simulink library "HANcoder_STM32_Target2009b"  (R2023a)
settings: Solver=ode45  StartTime=0.0  StopTime=10.0  RelTol=1e-3  EnableMultiTasking=on
libraries: simulink x3
(part 5 of 7)

== system HANcoder_STM32_Target2009b/STM32-P405/Timer Inputs ==
  Quadrature Encoder Get : Subsystem  Tag=HANcoder_TARGET_STM32_P405  mask(Quadrature Encoder Inputs){moduleID=TIM3: PORTC PIN6 & PORTC PIN7 - 5V Tolerant, config=Floating, counterReset=off, tsamp=-1}
      mask prompts: moduleID "Quad encoder module"; config "Configuration"; counterReset "Show counter reset input"; tsamp "Sample time"
      mask help:
      | Function
      | ========
      | Reads the counter of the quadrature encoder module.
      |
      | Parameters
      | ==========
      | Quadrature encoder module:
      |   Selects the quadrature encoder module. The channel A and B signals of the
      |   encoder should be connected to the 2 input pins that belong to the module.
      |
      | Configuration:
      |   Determines if the input is floating or is connected to an internal
      |   pull-up or pull-down resistor.
      |
      | Show counter reset input:
      |   Configures if the input port for the counter reset should be shown.
      |
      |
      | Outport
      | ==========
      | 32-bit signed counter. The counter starts at zero and counts up or down
      | depending on the direction of the motor.
      mask init:
      | moduleIDInfoStr = sfcn_quad_encoder_get_mcb(3,moduleID, counterReset, config);
      settings: CopyFcn=sfcn_quad_encoder_get_chk();  MoveFcn=drawLogos
      mask Help: web('sfcn_quad_encoder_get.html');
      mask TypeOptions moduleID: TIM1: PORTA PIN8 & PORTA PIN9 - 5V Tolerant | TIM3: PORTC PIN6 & PORTC PIN7 - 5V Tolerant | TIM4: PORTB PIN6 & PORTB PIN7 - 5V Tolerant
      mask Callback moduleID: sfcn_quad_encoder_get_chk();
      mask TypeOptions config: Floating | Pullup | Pulldown
      mask Display: fprintf('Quad Encoder Get\n%s', moduleIDInfoStr);patch([135 141 141],[8 14 2],[1 0 0]);patch([143 143 149],[14 2 8],[0 0 0.35]);
  Timer Input Get : Subsystem  Tag=HANcoder_TARGET_STM32_P405  mask(Timer Input Get){pin=TIM1: Con. PA8 (PORTA PIN8) - 5V Tolerant, zeroHzTimeoutMs=2000, tsamp=-1}
      mask prompts: pin "Timer input pin"; zeroHzTimeoutMs "0 Hz detection time (ms)"; tsamp "Sample time"
      mask help:
      | Function
      | ========
      | Reads the information from a timer input pin.
      |
      | Parameters
      | ==========
      | Timer input pin:
      |   Selects the timer input pin.
      |
      | Zero Hz detection time:
      |   Determines after how many milliseconds since the last edge the 0 Hz
      |   detected output flag should go high.
      |
      | Outport
      | ==========
      | Frequency
      |   The last measured frequency on the pin in Hz.
      |
      | Duty cycle
      |   The last measured duty cycle on the pin as a % with a scaling factor of 100 for
      |   improved resolution. So 5000 = 50% for example.
      |
      | Edge count
      |   The number of edges that were detected on the input pin since startup.
      |
      | Edge timestamp
      |   A 32-bit timestamp value of the last edge. The timestamp is derived from an
      |   internal 32-bit free running counter that runs at 21 Mhz.
      |
      | 0 Hz detected
      |   A boolean flag that will go high if no edges were detected for the time specified
      |   as the zero Hz detection time. Upon the next edge the flag will go low again.
      mask init:
      | timeinPinIdInfoStr = sfcn_timein_get_mcb(3, pin, zeroHzTimeoutMs);
      settings: CopyFcn=sfcn_timein_get_chk();  MoveFcn=drawLogos
      mask Help: web('sfcn_timein_get.html');
      mask TypeOptions pin: TIM1: Con. PA8 (PORTA PIN8) - 5V Tolerant | TIM1: Con. UEXT-3 (PORTA PIN9) - 5V Tolerant | TIM1: Con. UEXT-4 (PORTA PIN10) - 5V Tolerant | TIM2: Con. PA1 (PORTA PIN1) - 5V Tolerant | TIM3: Con. PC6 (PORTC PIN6) - 5V Tolerant | TIM3: Con. PC7 (PORTC PIN7) - 5V Tolerant | TIM3: Con. PC8 (PORTC PIN8) - 5V Tolerant | TIM3: Con. PC9 (PORTC PIN9) - 5V Tolerant | TIM4: Con. UEXT-5 (PORTB PIN6) - 5V Tolerant | TIM4: Con. UEXT-6 (PORTB PIN7) - 5V Tolerant | TIM4: Con. PB8 (PORTB PIN8) - 5V Tolerant | TIM4: Con. PB9 (PORTB PIN9) - 5V Tolerant
      mask Callback pin: sfcn_timein_get_chk();
      mask Display:
      | fprintf('Timer Input Get\n%s', timeinPinIdInfoStr);
      | port_label('output', 1, 'Frequency');
      | port_label('output', 2, 'Duty cycle');
      | port_label('output', 3, 'Edge count');
      | port_label('output', 4, 'Edge state');
      | port_label('output', 5, 'Edge timestamp');
      | port_label('output', 6, 'Counter timestamp');
      | port_label('output', 7, '0 Hz detected');patch([250 256 256],[8 14 2],[1 0 0]);patch([258 258 264],[14 2 8],[0 0 0.35]);
  Timer Input IRQ : Subsystem  Tag=HANcoder_TARGET_STM32_P405  mask(Timer Input IRQ){pin=TIM1: Con. PA8 (PORTA PIN8) - 5V Tolerant}
      mask prompts: pin "Timer input pin"
      mask help:
      | Function
      | ========
      | Enables a function call subsystem to be connected that is executed on interrupt level
      | each time an edge change on the input pin was detected.
      |
      | Parameters
      | ==========
      | Timer input pin:
      |   Selects the timer input pin.
      |
      | Outport
      | =======
      | IRQ
      |   Allows connection of a function call subsystem.
      mask init:
      | timeinPinIdInfoStr = sfcn_timein_irq_mcb(3, pin);
      settings: CopyFcn=sfcn_timein_irq_chk();  MoveFcn=drawLogos
      mask Help: web('sfcn_timein_irq.html');
      mask TypeOptions pin: TIM1: Con. PA8 (PORTA PIN8) - 5V Tolerant | TIM1: Con. UEXT-3 (PORTA PIN9) - 5V Tolerant | TIM1: Con. UEXT-4 (PORTA PIN10) - 5V Tolerant | TIM2: Con. PA1 (PORTA PIN1) - 5V Tolerant | TIM3: Con. PC6 (PORTC PIN6) - 5V Tolerant | TIM3: Con. PC7 (PORTC PIN7) - 5V Tolerant | TIM3: Con. PC8 (PORTC PIN8) - 5V Tolerant | TIM3: Con. PC9 (PORTC PIN9) - 5V Tolerant | TIM4: Con. UEXT-5 (PORTB PIN6) - 5V Tolerant | TIM4: Con. UEXT-6 (PORTB PIN7) - 5V Tolerant | TIM4: Con. PB8 (PORTB PIN8) - 5V Tolerant | TIM4: Con. PB9 (PORTB PIN9) - 5V Tolerant
      mask Callback pin: sfcn_timein_irq_chk();
      mask Display: fprintf('Timer Input IRQ\n%s', timeinPinIdInfoStr);patch([250 256 256],[8 14 2],[1 0 0]);patch([258 258 264],[14 2 8],[0 0 0.35]);

== system HANcoder_STM32_Target2009b/STM32-P405/Timer Outputs ==
  Compare Event IRQ : Subsystem  Tag=HANcoder_TARGET_STM32_P405  mask(Compare Event IRQ){pin=TIM1: Con. PA8 (PORTA PIN8) - 5V Tolerant}
      mask prompts: pin "Timer output pin"
      mask help:
      | Function
      | ========
      | Enables a function call subsystem to be connected that is executed on interrupt
      | level each time an output compare event was triggered.
      |
      | Parameters
      | ==========
      | Timer Output Pin:
      |   Selects the timer channel.
      |
      | Outport
      | =======
      | IRQ
      |   Allows connection of a function call subsystem.
      mask init:
      | timeoutPinIdInfoStr = sfcn_timeout_event_irq_mcb(3, pin);
      settings: CopyFcn=sfcn_timeout_event_irq_chk();  MoveFcn=drawLogos
      mask Help: web('sfcn_timeout_event_irq.html');
      mask TypeOptions pin: TIM1: Con. PA8 (PORTA PIN8) - 5V Tolerant | TIM1: Con. UEXT-3 (PORTA PIN9) - 5V Tolerant | TIM1: Con. UEXT-4 (PORTA PIN10) - 5V Tolerant | TIM2: Con. PA1 (PORTA PIN1) - 5V Tolerant | TIM3: Con. PC6 (PORTC PIN6) - 5V Tolerant | TIM3: Con. PC7 (PORTC PIN7) - 5V Tolerant | TIM3: Con. PC8 (PORTC PIN8) - 5V Tolerant | TIM3: Con. PC9 (PORTC PIN9) - 5V Tolerant | TIM4: Con. UEXT-5 (PORTB PIN6) - 5V Tolerant | TIM4: Con. UEXT-6 (PORTB PIN7) - 5V Tolerant | TIM4: Con. PB8 (PORTB PIN8) - 5V Tolerant | TIM4: Con. PB9 (PORTB PIN9) - 5V Tolerant
      mask Callback pin: sfcn_timeout_event_irq_chk();
      mask Display: fprintf('Compare Event IRQ\n%s', timeoutPinIdInfoStr);patch([135 141 141],[8 14 2],[1 0 0]);patch([143 143 149],[14 2 8],[0 0 0.35]);
  Get Free Running Counter : Subsystem  Tag=HANcoder_TARGET_STM32_P405  mask(Get Free Running Counter){moduleID=TIM1, tsamp=-1}
      mask prompts: moduleID "Timer module"; tsamp "Sample time"
      mask help:
      | Function
      | ========
      | Reads the timer module's internal 16-bit free running counter value.
      |
      | Parameters
      | ==========
      | Timer Module:
      |   Selects the timer module.
      |
      | Outport
      | =======
      | 16-bit free running counter value.
      mask init:
      | moduleIDInfoStr = sfcn_timeout_getrunningcounter_mcb(3, moduleID);
      settings: MoveFcn=drawLogos
      mask Help: web('sfcn_timeout_getrunningcounter.html');
      mask TypeOptions moduleID: TIM1 | TIM2 | TIM3 | TIM4
      mask Display: fprintf('Get Free Running Counter\n%s', moduleIDInfoStr);patch([135 141 141],[8 14 2],[1 0 0]);patch([143 143 149],[14 2 8],[0 0 0.35]);
  Get Last Event Counter : Subsystem  Tag=HANcoder_TARGET_STM32_P405  mask(Get Last Event Counter){pin=TIM1: Con. PA8 (PORTA PIN8) - 5V Tolerant, tsamp=-1}
      mask prompts: pin "Timer output pin"; tsamp "Sample time"
      mask help:
      | Function
      | ========
      | Reads the timer channel's timestamp of the 16-bit free running counter
      | value at which the last output compare event occurred.
      |
      | Parameters
      | ==========
      | Timer Output Pin:
      |   Selects the timer channel.
      |
      | Outport
      | =======
      | 16-bit free running counter timestamp of the last output compare event.
      mask init:
      | timeoutPinIdInfoStr = sfcn_timeout_getlasteventcounter_mcb(3, pin);
      settings: MoveFcn=drawLogos
      mask Help: web('sfcn_timeout_getlasteventcounter.html');
      mask TypeOptions pin: TIM1: Con. PA8 (PORTA PIN8) - 5V Tolerant | TIM1: Con. UEXT-3 (PORTA PIN9) - 5V Tolerant | TIM1: Con. UEXT-4 (PORTA PIN10) - 5V Tolerant | TIM2: Con. PA1 (PORTA PIN1) - 5V Tolerant | TIM3: Con. PC6 (PORTC PIN6) - 5V Tolerant | TIM3: Con. PC7 (PORTC PIN7) - 5V Tolerant | TIM3: Con. PC8 (PORTC PIN8) - 5V Tolerant | TIM3: Con. PC9 (PORTC PIN9) - 5V Tolerant | TIM4: Con. UEXT-5 (PORTB PIN6) - 5V Tolerant | TIM4: Con. UEXT-6 (PORTB PIN7) - 5V Tolerant | TIM4: Con. PB8 (PORTB PIN8) - 5V Tolerant | TIM4: Con. PB9 (PORTB PIN9) - 5V Tolerant
      mask Display: fprintf('Get Last Event Counter\n%s', timeoutPinIdInfoStr);patch([135 141 141],[8 14 2],[1 0 0]);patch([143 143 149],[14 2 8],[0 0 0.35]);
  Output Compare Init : Subsystem  Tag=HANcoder_TARGET_STM32_P405  mask(Output Compare Init){moduleID=TIM1: PA8 & PA9 & PA10 & n/a, frequency=2000000, enableIRQoutput=off}
      mask prompts: moduleID "Timer module"; frequency "Frequency (free running counter) [Hz]"; enableIRQoutput "Enable IRQ output"
      mask help:
      | Function
      | ========
      | Initializes the timer module to allow output compare functionality on the
      | module's channels.
      |
      | Parameters
      | ==========
      | Timer Module:
      |   Selects the timer module.
      |
      | Frequency:
      |   Frequency at which the 16-bit free running counter counts.
      |
      | Enable IRQ output
      |   Controls whether or not the IRQ output is available.
      |
      | Outport
      | =======
      | IRQ
      |   Allows connection of a function call subsystem for the free running
      |   counter overflow event.
      mask init:
      | moduleIDInfoStr = sfcn_timeout_init_mcb(3, moduleID, frequency, enableIRQoutput);
      settings: CopyFcn=sfcn_timeout_init_chk();  MoveFcn=drawLogos
      mask Help: web('sfcn_timeout_init.html');
      mask TypeOptions moduleID: TIM1: PA8 & PA9 & PA10 & n/a | TIM2: n/a & PA1 & n/a & n/a | TIM3: PC6 & PC7 & PC8 & PC9 | TIM4: PB6 & PB7 & PC8 & PB9
      mask Callback moduleID: sfcn_timeout_init_chk();
      mask Display: fprintf('Output Compare Init\n%s', moduleIDInfoStr);patch([135 141 141],[8 14 2],[1 0 0]);patch([143 143 149],[14 2 8],[0 0 0.35]);
  Reset Free Running Counter : Subsystem  Tag=HANcoder_TARGET_STM32_P405  mask(Reset Free Running Counter){moduleID=TIM1}
      mask prompts: moduleID "Timer module"
      mask help:
      | Function
      | ========
      | Resets the value of the timer module's 16-bit free running counter back to
      | 0.
      |
      | Triggerport
      | ===========
      | Connect the port to a trigger source to execute the block only when necessary.
      mask init:
      | moduleIDInfoStr = sfcn_timeout_resetcounter_mcb(3, moduleID);
      settings: MoveFcn=drawLogos
      mask Help: web('sfcn_timeout_resetcounter.html');
      mask TypeOptions moduleID: TIM1 | TIM2 | TIM3 | TIM4
      mask Display: fprintf('Reset Free Running Counter\n%s', moduleIDInfoStr);patch([132 138 138],[8 14 2],[1 0 0]);patch([140 140 146],[14 2 8],[0 0 0.35]);
  Schedule Compare Event : Subsystem  Tag=HANcoder_TARGET_STM32_P405  mask(Schedule Compare Event){pin=TIM1: Con. PA8 (PORTA PIN8) - 5V Tolerant, tsamp=-1}
      mask prompts: pin "Timer output pin"; tsamp "Sample time"
      mask help:
      | Function
      | ========
      | Schedules the next output compare event. The first input determines the
      | value of the timer module's 16-bit free running counter when the event
      | should trigger. The second input determines the action that should
      | be taken on the timer channel's pin.
      |
      | Parameters
      | ==========
      | Timer output pin:
      |   Selects the timer channel's pin.
      |
      | Inport
      | ======
      | Counter
      |   Value of the timer module's 16-bit free running counter at which the
      |   event should trigger.
      |
      | Action
      |   Action to take on the channel's pin when the event triggers:
      |   0: set output pin to logic low.
      |   1: set output pin to logic high.
      |   2: invert logic state of the outpin pin.
      |   3: do nothing to the output pin.
      mask init:
      | timeoutPinIdInfoStr = sfcn_timeout_scheduleevent_mcb(3, pin);
      settings: MoveFcn=drawLogos
      mask Help: web('sfcn_timeout_scheduleevent.html');
      mask TypeOptions pin: TIM1: Con. PA8 (PORTA PIN8) - 5V Tolerant | TIM1: Con. UEXT-3 (PORTA PIN9) - 5V Tolerant | TIM1: Con. UEXT-4 (PORTA PIN10) - 5V Tolerant | TIM2: Con. PA1 (PORTA PIN1) - 5V Tolerant | TIM3: Con. PC6 (PORTC PIN6) - 5V Tolerant | TIM3: Con. PC7 (PORTC PIN7) - 5V Tolerant | TIM3: Con. PC8 (PORTC PIN8) - 5V Tolerant | TIM3: Con. PC9 (PORTC PIN9) - 5V Tolerant | TIM4: Con. UEXT-5 (PORTB PIN6) - 5V Tolerant | TIM4: Con. UEXT-6 (PORTB PIN7) - 5V Tolerant | TIM4: Con. PB8 (PORTB PIN8) - 5V Tolerant | TIM4: Con. PB9 (PORTB PIN9) - 5V Tolerant
      mask Display: fprintf('Schedule Compare Event\n%s', timeoutPinIdInfoStr);patch([135 141 141],[8 14 2],[1 0 0]);patch([143 143 149],[14 2 8],[0 0 0.35]);

== system HANcoder_STM32_Target2009b/STM32-P405/UART ==
  UART init : Subsystem  Tag=HANcoder_TARGET_STM32_P405  mask(UART init){channel=UART1: Con. UEXT-3 & Con. UEXT-4 (PA9 & PA10), baudrate=19200, databits=8, parity=none, stopbits=1, txbufsize=32, rxbufsize=32, useStatusOut=off}
      mask prompts: baudrate "Baudrate (bit/s)"; txbufsize "Transmit buffer size"; rxbufsize "Receive buffer size"; useStatusOut "Use status output"
      mask help:
      | Function
      | ==========
      | Initialized a UART channel.
      |
      | Parameters per channel
      | ======================
      | - Select channel
      | - Select baudrate
      | - Select number of databits
      | - Select parity
      | - Select number of stopbits
      | - Configure the size of the transmit buffer
      | - Configure the size of the reception buffer
      | - Enable/disable the status output port
      mask init:
      | uartChannelInfoStr = sfcn_uart_init_mcb(3, channel, baudrate, databits, parity, stopbits, txbufsize, rxbufsize, useStatusOut);
      settings: CopyFcn=sfcn_uart_init_chk();  MoveFcn=drawLogos
      mask Help: web('sfcn_uart_init.html')
      mask TypeOptions channel: UART1: Con. UEXT-3 & Con. UEXT-4 (PA9 & PA10) | UART2: SUB D9 (PA2 & PA3)
      mask Callback channel: sfcn_uart_init_chk();
      mask TypeOptions baudrate: 300 | 600 | 1200 | 2400 | 4800 | 9600 | 19200 | 38400 | 57600 | 115200
      mask TypeOptions databits: 8 | 9
      mask TypeOptions parity: none | even | odd
      mask TypeOptions stopbits: 1 | 2
      mask Display: fprintf('UART init\n%s', uartChannelInfoStr);patch([236 242 242],[8 14 2],[1 0 0]);patch([244 244 250],[14 2 8],[0 0 0.35]);
  UART receive : Subsystem  Tag=HANcoder_TARGET_STM32_P405  mask(UART receive){channel=UART1: Con. UEXT-3 & Con. UEXT-4 (PA9 & PA10), useStatusOut=off, tsamp=-1}
      mask prompts: useStatusOut "Use status outport"; tsamp "Sample time"
      mask help:
      | Function
      | ==========
      | Reads a byte from the UART reception buffer.
      |
      | Parameters per channel
      | ======================
      | - Select channel
      | - Select if the status output should be enabled.
      |
      | Outputs
      | =======
      | - The value of the receive byte.
      | - When the status output is 0, the reception buffer was empty.
      mask init:
      | uartChannelInfoStr = sfcn_uart_receive_mcb(3, channel, useStatusOut);
      settings: MoveFcn=drawLogos
      mask Help: web('sfcn_uart_receive.html')
      mask TypeOptions channel: UART1: Con. UEXT-3 & Con. UEXT-4 (PA9 & PA10) | UART2: SUB D9 (PA2 & PA3)
      mask Display: fprintf('UART receive\n%s', uartChannelInfoStr);patch([240 246 246],[8 14 2],[1 0 0]);patch([248 248 254],[14 2 8],[0 0 0.35]);
  UART receive buffer status : Subsystem  Tag=HANcoder_TARGET_STM32_P405  mask(UART receive buffer status){channel=UART1: Con. UEXT-3 & Con. UEXT-4 (PA9 & PA10), tsamp=-1}
      mask prompts: tsamp "Sample time"
      mask help:
      | Function
      | ==========
      | Obtains the number of received bytes that are currently stored in the
      | reception buffer.
      |
      | Parameters per channel
      | ======================
      | - Select channel
      |
      | Outputs
      | ======
      | - The number of bytes currently stored in the reception buffer.
      mask init:
      | uartChannelInfoStr = sfcn_uart_receive_size_mcb(3, channel);
      settings: MoveFcn=drawLogos
      mask Help: web('sfcn_uart_receive_size.html')
      mask TypeOptions channel: UART1: Con. UEXT-3 & Con. UEXT-4 (PA9 & PA10) | UART2: SUB D9 (PA2 & PA3)
      mask Display: fprintf('UART receive buffer status\n%s', uartChannelInfoStr);patch([245 251 251],[8 14 2],[1 0 0]);patch([253 253 259],[14 2 8],[0 0 0.35]);
  UART send : Subsystem  Tag=HANcoder_TARGET_STM32_P405  mask(UART send){channel=UART1: Con. UEXT-3 & Con. UEXT-4 (PA9 & PA10), useStatusOut=off, tsamp=-1}
      mask prompts: useStatusOut "Use status outport"; tsamp "Sample time"
      mask help:
      | Function
      | ==========
      | Transmits a byte on the UART communication interface.
      |
      | Parameters per channel
      | ======================
      | - Select channel
      | - Select if the status output should be enabled.
      |
      | Inputs
      | ======
      | - The byte to send
      |
      | Outputs
      | =======
      | - When the status output is 0, the byte could not be transmitted. Probably
      |   because the transmit buffer was configured too small.
      mask init:
      | uartChannelInfoStr = sfcn_uart_send_mcb(3, channel, useStatusOut);
      settings: MoveFcn=drawLogos
      mask Help: web('sfcn_uart_send.html')
      mask TypeOptions channel: UART1: Con. UEXT-3 & Con. UEXT-4 (PA9 & PA10) | UART2: SUB D9 (PA2 & PA3)
      mask Display: fprintf('UART send\n%s', uartChannelInfoStr);patch([245 251 251],[8 14 2],[1 0 0]);patch([253 253 259],[14 2 8],[0 0 0.35]);

== system HANcoder_STM32_Target2009b/STM32-P405/UDS ==
  UDS Get Key : Subsystem  Tag=HANcoder_TARGET_STM32_P405  mask(UDS Get Key){tsamp=-1}
      mask prompts: tsamp "Sample time"
      mask help:
      | Function
      | ==========
      | Reads the 32-bit key value that was received from the UDS tester.
      |
      | Outport
      | =======
      |  - Key value that was received from the UDS tester.
      mask init:
      | sfcn_uds_get_key_mcb();
      settings: MoveFcn=drawLogos
      mask Help: web('sfcn_uds_get_key.html');
      mask Display: fprintf('UDS Get Key');patch([65 71 71],[8 14 2],[1 0 0]);patch([73 73 79],[14 2 8],[0 0 0.35]);
  UDS Get Seed : Subsystem  Tag=HANcoder_TARGET_STM32_P405  mask(UDS Get Seed){tsamp=-1}
      mask prompts: tsamp "Sample time"
      mask help:
      | Function
      | ==========
      | Reads the 32-bit seed value to be used in the seed/key unlock sequence.
      |
      | Outport
      | =======
      |  - Seed value to be used in the seed/key unlock sequence.
      mask init:
      | sfcn_uds_get_seed_mcb();
      settings: MoveFcn=drawLogos
      mask Help: web('sfcn_uds_get_seed.html');
      mask Display: fprintf('UDS Get Seed');patch([65 71 71],[8 14 2],[1 0 0]);patch([73 73 79],[14 2 8],[0 0 0.35]);
  UDS Get Seed Event : Subsystem  Tag=HANcoder_TARGET_STM32_P405  mask(UDS Get Seed Event){}
      mask help:
      | Function
      | ========
      | A 'UDS Get Seed Event' block is needed when the parameter 'UDS seed/key
      | required' is set to TRUE (checked) in the 'UDS Init' block.
      |
      | This block has a function call output that gets triggered during a seed/key
      | sequence, when the UDS module needs a seed. The connected subsystem should
      | contain a 'UDS Set Seed' block to give the seed back to the UDS module.
      |
      | Outport
      | =======
      | Event
      |   Allows connection of a function call subsystem.
      mask init:
      | sfcn_uds_get_seed_event_mcb();
      settings: MoveFcn=drawLogos
      mask Help: web('sfcn_uds_get_seed_event.html');
      mask Display: fprintf('UDS Get Seed Event');patch([95 101 101],[8 14 2],[1 0 0]);patch([103 103 109],[14 2 8],[0 0 0.35]);
  UDS Init : Subsystem  Tag=HANcoder_TARGET_STM32_P405  mask(UDS Init){canChannel=CAN 1, canTxId=hex2dec('7E8'), canRxId=hex2dec('7E0'), tpBlockSize=4, tpSTmin=40, tpRxBuffSize=64, udsTxBuffSize=64, udsUseSeedKey=off}
      mask prompts: canChannel "CAN channel"; canTxId "CAN transmit ID"; canRxId "CAN receive ID"; tpBlockSize "TP blocksize"; tpSTmin "TP STmin"; tpRxBuffSize "TP reception buffer size"; udsTxBuffSize "UDS transmit buffer size"; udsUseSeedKey "UDS seed/key required"
      mask help:
      | Function
      | ==========
      | Initializes the Unified Diagnostic Services (UDS) communication module.
      |
      | Parameters
      | ==========
      | CAN channel: The CAN channel to communicate on
      | CAN transmit ID: CAN identifier for ECU to Tester
      | CAN receive ID: CAN identifier for Tester to ECU
      | TP blocksize: Number of CF's to receive before sending a FC
      | TP STmin: Min separation time (ms) expected between CF's
      | TP reception buffer size: Size of the buffer for TP receptions
      | UDS transmit buffer size: Size of the buffer for UDS/TP transmissions
      | UDS seed/key required: Requires a seed/key unlock sequence
      mask init:
      | sfcn_uds_init_mcb(canChannel, canTxId, canRxId, tpBlockSize, tpSTmin, tpRxBuffSize, udsTxBuffSize, udsUseSeedKey);
      settings: MoveFcn=drawLogos
      mask Help: web('sfcn_uds_init.html');
      mask TypeOptions canChannel: CAN 1 | CAN 2
      mask TypeOptions tpBlockSize: 1 | 2 | 3 | 4 | 5 | 6 | 7 | 8 | 9 | 10 | 11 | 12 | 13 | 14 | 15 | 16 | 17 | 18 | 19 | 20 | 21 | 22 | 23 | 24 | 25 | 26 | 27 | 28 | 29 | 30 | 31 | 32 | 33 | 34 | 35 | 36 | 37 | 38 | 39 | 40 | 41 | 42 | 43 | 44 | 45 | 46 | 47 | 48 | 49 | 50 | 51 | 52 | 53 | 54 | 55 | 56 | 57 | 58 | 59 | 60 | 61 | 62 | 63 | 64 | 65 | 66 | 67 | 68 | 69 | 70 | 71 | 72 | 73 | 74 | 75 | 76 | 77 | 78 | 79 | 80 | 81 | 82 | 83 | 84 | 85 | 86 | 87 | 88 | 89 | 90 | 91 | 92 | 93 | 94 | 95 | 96 | 97 | 98 | 99 | 100 | 101 | 102 | 103 | 104 | 105 | 106 | 107 | 108 | 109 | 110 | 111 | 112 | 113 | 114 | 115 | 116 | 117 | 118 | 119 | 120 | 121 | 122 | 123 | 124 | 125 | 126 | 127 | 128 | 129 | 130 | 131 | 132 | 133 | 134 | 135 | 136 | 137 | 138 | 139 | 140 | 141 | 142 | 143 | 144 | 145 | 146 | 147 | 148 | 149 | 150 | 151 | 152 | 153 | 154 | 155 | 156 | 157 | 158 | 159 | 160 | 161 | 162 | 163 | 164 | 165 | 166 | 167 | 168 | 169 | 170 | 171 | 172 | 173 | 174 | 175 | 176 | 177 | 178 | 179 | 180 | 181 | 182 | 183 | 184 | 185 | 186 | 187 | 188 | 189 | 190 | 191 | 192 | 193 | 194 | 195 | 196 | 197 | 198 | 199 | 200 | 201 | 202 | 203 | 204 | 205 | 206 | 207 | 208 | 209 | 210 | 211 | 212 | 213 | 214 | 215 | 216 | 217 | 218 | 219 | 220 | 221 | 222 | 223 | 224 | 225 | 226 | 227 | 228 | 229 | 230 | 231 | 232 | 233 | 234 | 235 | 236 | 237 | 238 | 239 | 240 | 241 | 242 | 243 | 244 | 245 | 246 | 247 | 248 | 249 | 250 | 251 | 252 | 253 | 254 | 255
      mask TypeOptions tpSTmin: 1 | 2 | 3 | 4 | 5 | 6 | 7 | 8 | 9 | 10 | 11 | 12 | 13 | 14 | 15 | 16 | 17 | 18 | 19 | 20 | 21 | 22 | 23 | 24 | 25 | 26 | 27 | 28 | 29 | 30 | 31 | 32 | 33 | 34 | 35 | 36 | 37 | 38 | 39 | 40 | 41 | 42 | 43 | 44 | 45 | 46 | 47 | 48 | 49 | 50 | 51 | 52 | 53 | 54 | 55 | 56 | 57 | 58 | 59 | 60 | 61 | 62 | 63 | 64 | 65 | 66 | 67 | 68 | 69 | 70 | 71 | 72 | 73 | 74 | 75 | 76 | 77 | 78 | 79 | 80 | 81 | 82 | 83 | 84 | 85 | 86 | 87 | 88 | 89 | 90 | 91 | 92 | 93 | 94 | 95 | 96 | 97 | 98 | 99 | 100 | 101 | 102 | 103 | 104 | 105 | 106 | 107 | 108 | 109 | 110 | 111 | 112 | 113 | 114 | 115 | 116 | 117 | 118 | 119 | 120 | 121 | 122 | 123 | 124 | 125 | 126 | 127 | 128 | 129 | 130 | 131 | 132 | 133 | 134 | 135 | 136 | 137 | 138 | 139 | 140 | 141 | 142 | 143 | 144 | 145 | 146 | 147 | 148 | 149 | 150 | 151 | 152 | 153 | 154 | 155 | 156 | 157 | 158 | 159 | 160 | 161 | 162 | 163 | 164 | 165 | 166 | 167 | 168 | 169 | 170 | 171 | 172 | 173 | 174 | 175 | 176 | 177 | 178 | 179 | 180 | 181 | 182 | 183 | 184 | 185 | 186 | 187 | 188 | 189 | 190 | 191 | 192 | 193 | 194 | 195 | 196 | 197 | 198 | 199 | 200 | 201 | 202 | 203 | 204 | 205 | 206 | 207 | 208 | 209 | 210 | 211 | 212 | 213 | 214 | 215 | 216 | 217 | 218 | 219 | 220 | 221 | 222 | 223 | 224 | 225 | 226 | 227 | 228 | 229 | 230 | 231 | 232 | 233 | 234 | 235 | 236 | 237 | 238 | 239 | 240 | 241 | 242 | 243 | 244 | 245 | 246 | 247 | 248 | 249 | 250 | 251 | 252 | 253 | 254 | 255
      mask Display:
      | fprintf('UDS Init\n(CAN %x)', canChannel);
      | patch([65 71 71],[8 14 2],[1 0 0]);patch([73 73 79],[14 2 8],[0 0 0.35]);
  UDS Set Key Verfied : Subsystem  Tag=HANcoder_TARGET_STM32_P405  mask(UDS Set Key Verified){tsamp=-1}
      mask prompts: tsamp "Sample time"
      mask help:
      | Function
      | ========
      | Informs the UDS module whether or not the key received from the UDS tester
      | is valid.
      |
      | Inport
      | ======
      |  - Set to TRUE in case the key was valid, FALSE otherwise.
      mask init:
      | sfcn_uds_set_key_verified_mcb();
      settings: MoveFcn=drawLogos
      mask Help: web('sfcn_uds_set_key_verified.html');
      mask Display: fprintf('UDS Set Key\nVerified');patch([65 71 71],[8 14 2],[1 0 0]);patch([73 73 79],[14 2 8],[0 0 0.35]);
  UDS Set Seed : Subsystem  Tag=HANcoder_TARGET_STM32_P405  mask(UDS Set Seed){tsamp=-1}
      mask prompts: tsamp "Sample time"
      mask help:
      | Function
      | ==========
      | Sets the 32-bit seed value to be used in the seed/key unlock sequence.
      |
      | Inport
      | ======
      |  - Seed value to be used in the seed/key unlock sequence.
      mask init:
      | sfcn_uds_set_seed_mcb();
      settings: MoveFcn=drawLogos
      mask Help: web('sfcn_uds_set_seed.html');
      mask Display: fprintf('UDS Set Seed');patch([65 71 71],[8 14 2],[1 0 0]);patch([73 73 79],[14 2 8],[0 0 0.35]);
  UDS Verify Key Event : Subsystem  Tag=HANcoder_TARGET_STM32_P405  mask(UDS Verify Key Event){}
      mask help:
      | Function
      | ========
      | A 'UDS Verify Key Event' block is needed when the parameter 'UDS seed/key
      | required' is set to TRUE (checked) in the 'UDS Init' block.
      |
      | This block has a function call output that gets triggered during a seed/key
      | sequence, when the UDS module received a 32-bit key from the tester that
      | needs to be verified. The connected subsystem should contain a 'UDS Set Key
      | Verfied' block to inform the UDS module if the received key was correct.
      |
      | Outport
      | =======
      | Event
      |   Allows connection of a function call subsystem.
      mask init:
      | sfcn_uds_verify_key_event_mcb();
      settings: MoveFcn=drawLogos
      mask Help: web('sfcn_uds_verify_key_event.html');
      mask Display: fprintf('UDS Verify Key Event');patch([95 101 101],[8 14 2],[1 0 0]);patch([103 103 109],[14 2 8],[0 0 0.35]);

== system HANcoder_STM32_Target2009b/Olimexino STM32/Analog Inputs/Analog Input ==
  Level-2 M-file S-Function : M-S-Function  FunctionName=sfcn_analog_in  Parameters=tsamp, pinID
  Out1 : Outport
  wires:
  Level-2 M-file S-Function/1 -> Out1/1

== system HANcoder_STM32_Target2009b/Olimexino STM32/CAN/CAN ==
  CAN receive : Subsystem  Tag=HANcoder_TARGET_STM32_Olimexino  mask(CAN receive){canBus=CAN 1, outputNumber=1, dataType=uint8, byteOrder=off, tsamp=-1}
      mask prompts: canBus "CAN channel"; outputNumber "Output ports"; dataType "Output datatype"; byteOrder "Byte order: Checked = MSB first, unchecked = LSB first."; tsamp "Sample time"
      mask help:
      | Function
      | ==========
      | Receive the newest message from the specified CAN channel.
      |
      | Parameters
      | ==========
      | CAN channel:             The CAN channel to send the message on.
      | Output ports:             The amount of output ports
      | Output datatype:       The datatype of the output ports
      | Byte order:                 Select MSB or LSB first
      | Sample time:              -1 or divisible by base sample time [seconds]
      |
      | Input
      | ==========
      | Port 1:                       CAN ID(uint32) in hexadecimal ie: hex2dec('0a'),
      | to receive extended identifiers set the 32nd bit high (OR with 0x80000000)
      |
      | Output
      | ==========
      | Port 1:                       Checks for new message(int8)
      | Port 2..9                     Message data
      mask init:
      | sfcn_can_receive_mcb(canBus, outputNumber, dataType, byteOrder)
      settings: MoveFcn=drawLogos
      mask Help: web('sfcn_can_receive.html');
      mask TypeOptions canBus: CAN 1
      mask TypeOptions dataType: int8 | uint8 | int16 | uint16 | int32 | uint32 | boolean
      mask Display:
      | fprintf('Receive on\nCAN %x', canBus);
      | port_label('output', 1, 'new')
      | port_label('input', 1, 'ID');patch([75 81 81],[8 14 2],[1 0 0]);patch([83 83 89],[14 2 8],[0 0 0.35]);
  CAN receive packed : Subsystem  Tag=HANcoder_TARGET_STM32_Olimexino  mask(CAN receive packed){canBus=CAN 1, canID=hex2dec('80'), tsamp=-1}
      mask prompts: canBus "CAN channel"; canID "Can ID (in hex)"; tsamp "Sample time"
      mask help:
      | Function
      | ==========
      | Receive the newest message from the specified CAN channel, packed in a CAN message signal.
      | The first output checks the receiving of new data.
      |
      | CAN channel: The specified CAN channel will be used to receive the message on.
      |
      | CAN ID (in hex): Only the message with the specified CAN identifier (ID) is received. The ID is written in hexadecimal format, ie: hex2dec('0A')
      |
      | PS. No data is unpacked by the 'CAN Unpack' block when the data output is directly connected to a terminator (an example, placing a *1 'Gain' in between will solve this).
      mask init:
      | sfcn_can_receive_packed_mcb(canBus, canID)
      settings: MoveFcn=drawLogos
      mask Help: web('sfcn_can_receive_packed.html');
      mask TypeOptions canBus: CAN 1
      mask Display: fprintf('Receive packed CAN\nmessage on CAN %x\nID %xh', canBus, canID);patch([95 101 101],[8 14 2],[1 0 0]);patch([103 103 109],[14 2 8],[0 0 0.35]);
  CAN send : Subsystem  Tag=HANcoder_TARGET_STM32_Olimexino  mask(CAN send){canBus=CAN 1, frameType=Standard (11 bit), inputNumber=8, dataType=uint8, byteOrder=on, tsamp=-1}
      mask prompts: canBus "CAN channel"; frameType "Identifier type"; inputNumber "Input ports"; dataType "Input datatype"; byteOrder "Byte order: Checked = MSB first, unchecked = LSB first."; tsamp "Sample time"
      mask help:
      | Function
      | ==========
      | Send a message on the CAN channel.
      |
      | Parameters
      | ==========
      | CAN channel:           The CAN channel to send the message on.
      | Identifier type:         normal or extended ID's
      | Input ports:              The amount of input ports
      | Input datatype:        The datatype of the input ports
      | Byte order:               Select MSB or LSB first
      | Sample time:            -1 or divisible by base sample time [seconds]
      |
      | Input
      | ==========
      | Port 1:                   CAN ID(uint32) in hexadecimal ie: hex2dec('0a')
      | Port 2..9                CAN message data
      mask init:
      | sfcn_can_send_mcb(canBus, frameType, inputNumber, dataType, byteOrder)
      settings: MoveFcn=drawLogos
      mask Help: web('sfcn_can_send.html');
      mask TypeOptions canBus: CAN 1
      mask TypeOptions frameType: Standard (11 bit) | Extended (29 bit)
      mask TypeOptions dataType: int8 | uint8 | int16 | uint16 | int32 | uint32 | boolean
      mask Display:
      | fprintf('Send on\nCAN %x', canBus);
      | port_label('input', 1, 'ID');patch([65 71 71],[8 14 2],[1 0 0]);patch([73 73 79],[14 2 8],[0 0 0.35]);
  CAN send packed : Subsystem  Tag=HANcoder_TARGET_STM32_Olimexino  mask(CAN send packed){canBus=CAN 1, tsamp=-1}
      mask prompts: canBus "CAN channel"; tsamp "Sample time"
      mask help:
      | Function
      | ==========
      | Send a packed CAN message on the specified CAN channel.
      |
      | CAN channel: The specified CAN channel will be used to send the message on.
      |
      | The CAN ID, identifier type and formatting of the data is included in the packed CAN message.
      mask init:
      | sfcn_can_send_packed_mcb(canBus)
      settings: MoveFcn=drawLogos
      mask Help: web('sfcn_can_send_packed.html');
      mask TypeOptions canBus: CAN 1
      mask Display: fprintf('Send packed CAN\n message on CAN %x', canBus);patch([95 101 101],[8 14 2],[1 0 0]);patch([103 103 109],[14 2 8],[0 0 0.35]);

== system HANcoder_STM32_Target2009b/Olimexino STM32/CAN/CANopenNode ==
  CANopenNode Init : Subsystem  Tag=HANcoder_TARGET_STM32_Olimexino  mask(CANopenNode Init){channel=CAN 1}
      mask prompts: channel "CAN channel"
      mask help:
      | Function
      | ==========
      | Initializes the CANopenNode stack for the particular CAN channel.
      |
      | CAN channel: The specified CAN channel will be used by the communication stack.
      mask init:
      | sfcn_can_canopennode_init_mcb(channel)
      settings: MoveFcn=drawLogos
      mask Help: web('sfcn_can_canopennode_init.html');
      mask TypeOptions channel: CAN 1
      mask Display: fprintf('CANopenNode\n Init on CAN %d', channel);patch([95 101 101],[8 14 2],[1 0 0]);patch([103 103 109],[14 2 8],[0 0 0.35]);
  CANopenNode OD Read : Subsystem  Tag=HANcoder_TARGET_STM32_Olimexino  mask(CANopenNode OD Read){index=hex2dec('6200'), subIndex=1, dataType=uint8, tsamp=-1}
      mask prompts: index "OD index"; subIndex "OD subindex"; dataType "OD data type"; tsamp "Sample time"
      mask help:
      | Function
      | ==========
      | Reads a data value from the internal object dictionary.
      |
      | OD Index: Index of the object dictionary to read from.
      | OD Subindex: Subindex of the object dictionary to read from.
      | OD Data type: Data type of the object dictionary to read from.
      mask init:
      | sfcn_can_canopennode_od_read_mcb(index, subIndex, dataType)
      settings: MoveFcn=drawLogos
      mask Help: web('sfcn_can_canopennode_od_read.html');
      mask TypeOptions dataType: int8 | uint8 | int16 | uint16 | int32 | uint32
      mask Display: fprintf('CANopenNode\n OD Read\nindex: 0x%x\nsubindex: %d', index, subIndex');patch([95 101 101],[8 14 2],[1 0 0]);patch([103 103 109],[14 2 8],[0 0 0.35]);
  CANopenNode OD Write : Subsystem  Tag=HANcoder_TARGET_STM32_Olimexino  mask(CANopenNode OD Write){index=hex2dec('6000'), subIndex=1, dataType=uint8, tsamp=-1}
      mask prompts: index "OD index"; subIndex "OD subindex"; dataType "OD data type"; tsamp "Sample time"
      mask help:
      | Function
      | ==========
      | Writes a data value to the internal object dictionary.
      |
      | OD Index: Index of the object dictionary to write to.
      | OD Subindex: Subindex of the object dictionary to write to.
      | OD Data type: Data type of the object dictionary to write to.
      mask init:
      | sfcn_can_canopennode_od_write_mcb(index, subIndex, dataType)
      settings: MoveFcn=drawLogos
      mask Help: web('sfcn_can_canopennode_od_write.html');
      mask TypeOptions dataType: int8 | uint8 | int16 | uint16 | int32 | uint32
      mask Display: fprintf('CANopenNode\n OD Write\nindex: 0x%x\nsubindex: %d', index, subIndex);patch([95 101 101],[8 14 2],[1 0 0]);patch([103 103 109],[14 2 8],[0 0 0.35]);

== system HANcoder_STM32_Target2009b/Olimexino STM32/Digital Inputs/Digital Input ==
  Level-2 M-file S-Function : M-S-Function  FunctionName=sfcn_digital_in  Parameters=tsamp, pinID, config
  Out1 : Outport
  wires:
  Level-2 M-file S-Function/1 -> Out1/1

== system HANcoder_STM32_Target2009b/Olimexino STM32/Digital Outputs/Digital Output ==
  In1 : Inport
  Level-2 M-file S-Function : M-S-Function  FunctionName=sfcn_digital_out  Parameters=tsamp, pinID, config
  wires:
  In1/1 -> Level-2 M-file S-Function/1

== system HANcoder_STM32_Target2009b/Olimexino STM32/Error Handling/Clear errors ==
  Trigger : TriggerPort  VariantControl=(inherit)
  Level-2 M-file S-Function : M-S-Function  FunctionName=sfcn_controller_error_clearerrors  Parameters=eepromString

== system HANcoder_STM32_Target2009b/Olimexino STM32/Error Handling/Delete error ==
  Trigger : TriggerPort  VariantControl=(inherit)
  Constant : Constant  OutDataTypeStr=uint8  SampleTime=-1
  Gnd1 : Ground
  Gnd2 : Ground
  Level-2 M-file S-Function : M-S-Function  FunctionName=sfcn_controller_error_deleteerror_in  Parameters=useInPorts, errorID, para
  wires:
  Gnd2/1 -> Level-2 M-file S-Function/2
  Gnd1/1 -> Level-2 M-file S-Function/1
  Constant/1 -> Level-2 M-file S-Function/3

== system HANcoder_STM32_Target2009b/Olimexino STM32/Error Handling/Read active error ==
  In1 : Inport
  Level-2 M-file S-Function : M-S-Function  FunctionName=sfcn_controller_error_readerror  Parameters=tsamp
  numbers : Outport
  code : Outport  Port=2
  parameter : Outport  Port=3
  Xtimes : Outport  Port=4
  timestamp : Outport  Port=5
  wires:
  Level-2 M-file S-Function/1 -> numbers/1
  Level-2 M-file S-Function/2 -> code/1
  Level-2 M-file S-Function/3 -> parameter/1
  Level-2 M-file S-Function/4 -> Xtimes/1
  Level-2 M-file S-Function/5 -> timestamp/1
  In1/1 -> Level-2 M-file S-Function/1

== system HANcoder_STM32_Target2009b/Olimexino STM32/Error Handling/Read stored error ==
  In1 : Inport
  Level-2 M-file S-Function : M-S-Function  FunctionName=sfcn_controller_error_readerror  Parameters=tsamp
  numbers : Outport
  code : Outport  Port=2
  parameter : Outport  Port=3
  Xtimes : Outport  Port=4
  timestamp : Outport  Port=5
  wires:
  In1/1 -> Level-2 M-file S-Function/1
  Level-2 M-file S-Function/5 -> timestamp/1
  Level-2 M-file S-Function/4 -> Xtimes/1
  Level-2 M-file S-Function/3 -> parameter/1
  Level-2 M-file S-Function/2 -> code/1
  Level-2 M-file S-Function/1 -> numbers/1

== system HANcoder_STM32_Target2009b/Olimexino STM32/Error Handling/Search active error ==
  In1 : Inport
  In2 : Inport  Port=2
  Level-2 M-file S-Function : M-S-Function  FunctionName=sfcn_controller_error_searcherror  Parameters=tsamp
  occurrence : Outport
  timestamp : Outport  Port=2
  wires:
  In1/1 -> Level-2 M-file S-Function/1
  In2/1 -> Level-2 M-file S-Function/2
  Level-2 M-file S-Function/1 -> occurrence/1
  Level-2 M-file S-Function/2 -> timestamp/1

== system HANcoder_STM32_Target2009b/Olimexino STM32/Error Handling/Search stored error ==
  In1 : Inport
  In2 : Inport  Port=2
  Level-2 M-file S-Function : M-S-Function  FunctionName=sfcn_controller_error_searcherror  Parameters=tsamp
  occurrence : Outport
  timestamp : Outport  Port=2
  wires:
  Level-2 M-file S-Function/2 -> timestamp/1
  Level-2 M-file S-Function/1 -> occurrence/1
  In2/1 -> Level-2 M-file S-Function/2
  In1/1 -> Level-2 M-file S-Function/1

== system HANcoder_STM32_Target2009b/Olimexino STM32/Error Handling/Store error  ==
  Trigger : TriggerPort  VariantControl=(inherit)
  Gnd1 : Ground
  Gnd2 : Ground
  Level-2 M-file S-Function : M-S-Function  FunctionName=sfcn_controller_error_storeerror_in  Parameters=useInPorts, errorCode, parameter
  wires:
  Gnd1/1 -> Level-2 M-file S-Function/1
  Gnd2/1 -> Level-2 M-file S-Function/2

== system HANcoder_STM32_Target2009b/Olimexino STM32/Error Handling/Total Errors ==
  Level-2 M-file S-Function : M-S-Function  FunctionName=sfcn_controller_error_totalerrors  Parameters=eepromString, tsamp
  Out1 : Outport
  Out2 : Outport  Port=2
  wires:
  Level-2 M-file S-Function/1 -> Out1/1
  Level-2 M-file S-Function/2 -> Out2/1

== system HANcoder_STM32_Target2009b/Olimexino STM32/File Logger/File Logger Close ==
  Trigger : TriggerPort  VariantControl=(inherit)
  Level-2 M-file S-Function : M-S-Function  FunctionName=sfcn_filelogger_close

== system HANcoder_STM32_Target2009b/Olimexino STM32/File Logger/File Logger Init ==
  (Re)start : TriggerPort  VariantControl=(inherit)
  Level-2 M-file S-Function : M-S-Function  FunctionName=sfcn_filelogger_init

== system HANcoder_STM32_Target2009b/Olimexino STM32/File Logger/File Logger Signal ==
  In1 : Inport
  Level-2 M-file S-Function : M-S-Function  FunctionName=sfcn_filelogger_signal  Parameters=dataType
  wires:
  In1/1 -> Level-2 M-file S-Function/1

== system HANcoder_STM32_Target2009b/Olimexino STM32/Memory/EEPROM ==
  Erase EEPROM : Subsystem  Tag=HANcoder_TARGET_STM32_Olimexino  mask(Erase EEPROM){}
      mask help:
      | Function
      | ========
      | Erases all identifier values from EEPROM.
      |
      | Triggerport
      | ===========
      | Connect the port to a trigger source to execute the block only when necessary.
      mask init:
      | sfcn_eeprom_clear_mcb();
      settings: MoveFcn=drawLogos
      mask Display: fprintf('Erase EEPROM');patch([80 86 86],[8 14 2],[1 0 0]);patch([88 88 94],[14 2 8],[0 0 0.35]);
  Read from EEPROM : Subsystem  Tag=HANcoder_TARGET_STM32_Olimexino  mask(Read from EEPROM){tsamp=-1}
      mask prompts: tsamp "Sample time"
      mask help:
      | Function
      | ========
      | Read a value from the specified EEPROM identifier.
      |
      | Inport
      | ==========
      | id:
      |   The EEPROM identifier. This input is of type UINT8 and can have a value
      |   between 0..255 to select one of the 256 supported application specific
      |   identifiers.
      |
      | Outport
      | =======
      | value:
      |   The value read from the EEPROM identifier. This output is of type UINT16.
      mask init:
      | sfcn_eeprom_read_mcb();
      settings: MoveFcn=drawLogos
      mask Display:
      | fprintf('Read from EEPROM');
      | port_label('input', 1, 'id');
      | port_label('output', 1, 'value');patch([150 156 156],[8 14 2],[1 0 0]);patch([158 158 164],[14 2 8],[0 0 0.35]);
  Save EEPROM : Subsystem  Tag=HANcoder_TARGET_STM32_Olimexino  mask(Save EEPROM){}
      mask help:
      | Function
      | ========
      | The STM32 controller does not have dedicated EEPROM on-chip. All EEPROM
      | write, read and erase operations are therefore performed in a RAM buffer.
      | To make sure RAM buffer contents are still valid after a power-off, its
      | contents needs to be save in flash EEPROM, which is achieved with this
      | block. This is typically called during the software shutdown sequence,
      | right before power off.
      |
      | Triggerport
      | ===========
      | Connect the port to a trigger source to execute the block only when necessary.
      mask init:
      | sfcn_eeprom_save_mcb();
      settings: MoveFcn=drawLogos
      mask Display: fprintf('Save EEPROM');patch([80 86 86],[8 14 2],[1 0 0]);patch([88 88 94],[14 2 8],[0 0 0.35]);
  Write to EEPROM : Subsystem  Tag=HANcoder_TARGET_STM32_Olimexino  mask(Write to EEPROM){tsamp=-1}
      mask prompts: tsamp "Sample time"
      mask help:
      | Function
      | ========
      | Write the value to the specified EEPROM identifier.
      |
      | Inport
      | ==========
      | id:
      |   The EEPROM identifier. This input is of type UINT8 and can have a value
      |   between 0..255 to select one of the 256 supported application specific
      |   identifiers.
      | value:
      |   The value to write to the EEPROM identifier. This input is of type UINT16.
      mask init:
      | sfcn_eeprom_write_mcb();
      settings: MoveFcn=drawLogos
      mask Display:
      | fprintf('Write to EEPROM');
      | port_label('input', 1, 'id');
      | port_label('input', 2, 'value');patch([150 156 156],[8 14 2],[1 0 0]);patch([158 158 164],[14 2 8],[0 0 0.35]);

== system HANcoder_STM32_Target2009b/Olimexino STM32/PWM Outputs/PWM Duty Cycle ==
  In1 : Inport
  Level-2 M-file S-Function : M-S-Function  FunctionName=sfcn_pwmout_setduty  Parameters=tsamp
  wires:
  In1/1 -> Level-2 M-file S-Function/1

== system HANcoder_STM32_Target2009b/Olimexino STM32/PWM Outputs/PWM Init ==
  S-Function : S-Function  FunctionName=sfcn_pwmout_init  SFunctionDeploymentMode=off  EnableBusSupport=off
  Term1 : Terminator
  wires:
  S-Function/1 -> Term1/1

== system HANcoder_STM32_Target2009b/Olimexino STM32/SPI/SPI master init ==
  Level-2 M-file S-Function : M-S-Function  FunctionName=sfcn_spi_master_init

== system HANcoder_STM32_Target2009b/Olimexino STM32/SPI/SPI master transfer ==
  In1 : Inport
  Level-2 M-file S-Function : M-S-Function  FunctionName=sfcn_spi_master_transfer  Parameters=tsamp
  Out1 : Outport
  wires:
  In1/1 -> Level-2 M-file S-Function/1
  Level-2 M-file S-Function/1 -> Out1/1

== system HANcoder_STM32_Target2009b/Olimexino STM32/System Config/Base Sample Time config ==
  note: This constant and terminator block introduces the base sample time,
      | set in Base Sample Time config block, to the model. Blocks  with inherited [-1]
      | sample time wich are not connected to blocks with specifically set sample times
      | will use this value. This block also sets the fixed step time parameter in the Simulink Solver.
      | This works during initialization of simulation or build.
  Level-2 M-file S-Function : M-S-Function  FunctionName=sfcn_base_sample_time  Parameters=baseSampleTime, extraStack
  SampleTimeCrowBar : Constant  InitFcn=|  VectorParams1D=off  OutDataTypeStr=boolean  SampleTime=0.01
      | SampleTimeMiliSeconds = get_param(find_system(bdroot, 'LookUnderMasks', 'all', 'FollowLinks', 'off',  'Name', 'Base Sample Time config'), 'baseSampleTime');
      |                                                                                                                                                             
      | SampleTimeSeconds = str2num(SampleTimeMiliSeconds{1,1})/1000;                                                                                               
      |                                                                                                                                                             
      | set_param(bdroot, 'FixedStep', num2str(SampleTimeSeconds));                                                                                                 
      |                                                                                                                                                             
      | set_param(gcb, 'SampleTime', num2str(get_param(bdroot, 'FixedStep')));                                                                                      
      | clear SampleTimeSeconds SampleTimeMiliSeconds
  Terminator : Terminator
  wires:
  SampleTimeCrowBar/1 -> Terminator/1

== system HANcoder_STM32_Target2009b/Olimexino STM32/System Config/Build settings ==

== system HANcoder_STM32_Target2009b/Olimexino STM32/System Config/CAN config ==
  Level-2 M-file S-Function : M-S-Function  FunctionName=sfcn_can_config

== system HANcoder_STM32_Target2009b/Olimexino STM32/System Config/Custom ID config ==
  Level-2 M-file S-Function : M-S-Function  RequirementInfo={}  FunctionName=sfcn_custom_version_config  Parameters=softID

== system HANcoder_STM32_Target2009b/Olimexino STM32/System Config/XCP on CAN config ==
  Level-2 M-file S-Function : M-S-Function  RequirementInfo={} %GIDa_75ebdf1d_e085_4bd4_9cf7_36846954f0a6  FunctionName=sfcn_can_xcp_config  Parameters=canBus, croID, dtoID

== system HANcoder_STM32_Target2009b/Olimexino STM32/System Config/XCP on USB config ==
  Level-2 M-file S-Function : M-S-Function  RequirementInfo={} %GIDa_75ebdf1d_e085_4bd4_9cf7_36846954f0a6  FunctionName=sfcn_usb_xcp_config

== system HANcoder_STM32_Target2009b/Olimexino STM32/System Management/Enter Critical Section ==
  Level-2 M-file S-Function : M-S-Function  FunctionName=sfcn_critical_enter  Parameters=tsamp

== system HANcoder_STM32_Target2009b/Olimexino STM32/System Management/Exit Critical Section ==
  Level-2 M-file S-Function : M-S-Function  FunctionName=sfcn_critical_exit  Parameters=tsamp

== system HANcoder_STM32_Target2009b/Olimexino STM32/System Management/Get CPU load ==
  Level-2 M-file S-Function : M-S-Function  FunctionName=sfcn_controller_cpu_getload  Parameters=tsamp, mode
  Out1 : Outport
  wires:
  Level-2 M-file S-Function/1 -> Out1/1

== system HANcoder_STM32_Target2009b/Olimexino STM32/System Management/Get free Heap ==
  Level-2 M-file S-Function : M-S-Function  FunctionName=sfcn_controller_getheap  Parameters=tsamp
  Out1 : Outport
  wires:
  Level-2 M-file S-Function/1 -> Out1/1

== system HANcoder_STM32_Target2009b/Olimexino STM32/System Management/Get free Stack ==
  Level-2 M-file S-Function : M-S-Function  FunctionName=sfcn_controller_getstack  Parameters=tsamp, taskIdx
  Out1 : Outport
  wires:
  Level-2 M-file S-Function/1 -> Out1/1

== system HANcoder_STM32_Target2009b/Olimexino STM32/System Management/Reset ECU ==
  Trigger : TriggerPort  VariantControl=(inherit)
  Level-2 M-file S-Function : M-S-Function  FunctionName=sfcn_controller_reset

== system HANcoder_STM32_Target2009b/Olimexino STM32/Timer Inputs/Quadrature Encoder Get ==
  Data Type Conversion : DataTypeConversion  OutDataTypeStr=boolean  SaturateOnIntegerOverflow=off  RndMeth=Floor
  Detect Increase : simulink/Logic and Bit Operations/Detect Increase  vinit=0.0  OutDataTypeStr=uint8
  Gnd1 : Ground
  Level-2 M-file S-Function : M-S-Function  FunctionName=sfcn_quad_encoder_get  Parameters=tsamp, moduleID
  Out1 : Outport
  wires:
  Level-2 M-file S-Function/1 -> Out1/1
  Gnd1/1 -> Detect Increase/1
  Detect Increase/1 -> Data Type Conversion/1
  Data Type Conversion/1 -> Level-2 M-file S-Function/1

== system HANcoder_STM32_Target2009b/Olimexino STM32/Timer Inputs/Timer Input Get ==
  Level-2 M-file S-Function : M-S-Function  FunctionName=sfcn_timein_get  Parameters=tsamp
  Out1 : Outport
  Out2 : Outport  Port=2
  Out3 : Outport  Port=3
  Out4 : Outport  Port=4
  Out5 : Outport  Port=5
  Out6 : Outport  Port=6
  Out7 : Outport  Port=7
  wires:
  Level-2 M-file S-Function/1 -> Out1/1
  Level-2 M-file S-Function/2 -> Out2/1
  Level-2 M-file S-Function/3 -> Out3/1
  Level-2 M-file S-Function/4 -> Out4/1
  Level-2 M-file S-Function/5 -> Out5/1
  Level-2 M-file S-Function/6 -> Out6/1
  Level-2 M-file S-Function/7 -> Out7/1

== system HANcoder_STM32_Target2009b/Olimexino STM32/Timer Inputs/Timer Input IRQ ==
  S-Function : S-Function  FunctionName=sfcn_timein_irq  SFunctionDeploymentMode=off  EnableBusSupport=off
  Out1 : Outport
  wires:
  S-Function/1 -> Out1/1

== system HANcoder_STM32_Target2009b/Olimexino STM32/Timer Outputs/Compare Event IRQ ==
  S-Function : S-Function  FunctionName=sfcn_timeout_event_irq  SFunctionDeploymentMode=off  EnableBusSupport=off
  Out1 : Outport
  wires:
  S-Function/1 -> Out1/1

== system HANcoder_STM32_Target2009b/Olimexino STM32/Timer Outputs/Get Free Running Counter ==
  Level-2 M-file S-Function : M-S-Function  FunctionName=sfcn_timeout_getrunningcounter  Parameters=tsamp
  Out1 : Outport
  wires:
  Level-2 M-file S-Function/1 -> Out1/1

== system HANcoder_STM32_Target2009b/Olimexino STM32/Timer Outputs/Get Last Event Counter ==
  Level-2 M-file S-Function : M-S-Function  FunctionName=sfcn_timeout_getlasteventcounter  Parameters=tsamp
  Out1 : Outport
  wires:
  Level-2 M-file S-Function/1 -> Out1/1

== system HANcoder_STM32_Target2009b/Olimexino STM32/Timer Outputs/Output Compare Init ==
  S-Function : S-Function  FunctionName=sfcn_timeout_init  SFunctionDeploymentMode=off  EnableBusSupport=off
  Term1 : Terminator
  wires:
  S-Function/1 -> Term1/1
